simulink model "chaotic_freq_spring_multfeedback"  (Simulink 7.8)
settings: Solver=ode4  StartTime=h  StopTime=2000  FixedStep=h  RelTol=1e-3
undefined symbols (not defined in the file): a, b, c, k, tau, w
settings Model: Creator=stepp  LastModifiedBy=stepp  ExtModeAutoUpdateStatusClock=off
settings DataIOCC: LimitDataPoints=off  SaveState=on  SignalLogging=off  StateSaveName=x  TimeSaveName=t  OutputSaveName=y
settings OptimizationCC: InitFltsAndDblsToZero=on
settings DebuggingCC: SaveWithParameterizedLinksMsg=none  StrictBusMsg=Warning
settings GRTTargetCC: TargetFcnLib=ansi_tfl_tmw.mat

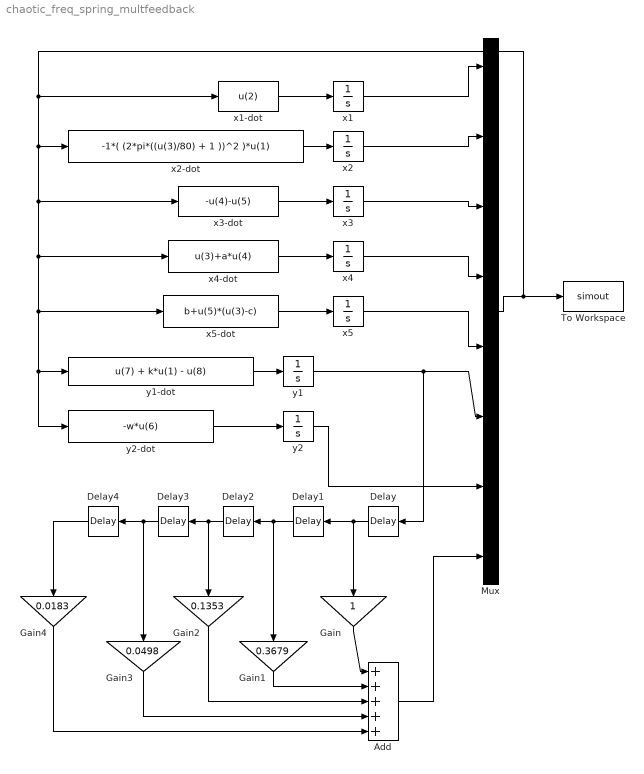
== system chaotic_freq_spring_multfeedback ==
  Add : Sum  Inputs=5
  Delay{,1..4} (5 alike) : TransportDelay  DelayTime=tau
  Gain : Gain
  Gain1 : Gain  Gain=0.3679
  Gain2 : Gain  Gain=0.1353
  Gain3 : Gain  Gain=0.0498
  Gain4 : Gain  Gain=0.0183
  Mux : Mux  Inputs=8
  To Workspace : ToWorkspace  VariableName=simout  SampleTime=-1  SaveFormat=Array
  x1 : Integrator  InitialCondition=1
  x1-dot : Fcn  Expr=u(2)
  x2 : Integrator
  x2-dot : Fcn  Expr=-1*( (2*pi*((u(3)/80) + 1 ))^2 )*u(1)
  x3 : Integrator  InitialCondition=18.68
  x3-dot : Fcn  Expr=-u(4)-u(5)
  x4 : Integrator  InitialCondition=3.432
  x4-dot : Fcn  Expr=u(3)+a*u(4)
  x5 : Integrator  InitialCondition=20.9
  x5-dot : Fcn  Expr=b+u(5)*(u(3)-c)
  y1 : Integrator  InitialCondition=1
  y1-dot : Fcn  Expr=u(7) + k*u(1) - u(8)
  y2 : Integrator
  y2-dot : Fcn  Expr=-w*u(6)
  wires:
  x1-dot/1 -> x1/1
  x2-dot/1 -> x2/1
  x3-dot/1 -> x3/1
  x4-dot/1 -> x4/1
  x5-dot/1 -> x5/1
  x1/1 -> Mux/1
  x2/1 -> Mux/2
  x3/1 -> Mux/3
  x4/1 -> Mux/4
  x5/1 -> Mux/5
  Mux/1 -> x1-dot/1, x2-dot/1, x3-dot/1, x4-dot/1, x5-dot/1, y1-dot/1, y2-dot/1, To Workspace/1
  y2-dot/1 -> y2/1
  y1-dot/1 -> y1/1
  y1/1 -> Delay/1, Mux/6
  y2/1 -> Mux/7
  Delay/1 -> Delay1/1, Gain/1
  Delay1/1 -> Delay2/1, Gain1/1
  Delay2/1 -> Delay3/1, Gain2/1
  Add/1 -> Mux/8
  Delay3/1 -> Delay4/1, Gain3/1
  Delay4/1 -> Gain4/1
  Gain/1 -> Add/1
  Gain1/1 -> Add/2
  Gain2/1 -> Add/3
  Gain3/1 -> Add/4
  Gain4/1 -> Add/5
